simulink model "codec74"  (R2018a)
settings: Solver=VariableStepAuto  StartTime=0.0  StopTime=10.0  RelTol=1e-3
values from neighbouring files (symbols this model uses):
  pbsc74 = i    [Ejercicio44.m]
libraries: commblkcod2 x2, commrandsrc3 x1, commchan3 x1, commsink2 x1
settings Model: Creator=Alumnos  LastModifiedBy=Anselmo-PC

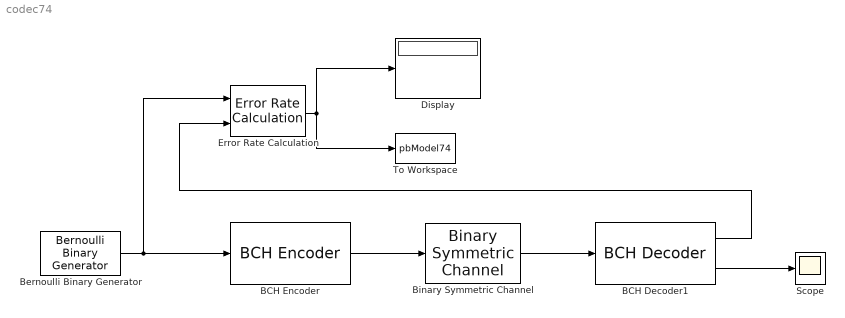
== system codec74 ==
  BCH Decoder1 : commblkcod2/BCH Decoder  n=7  k=4  specShortening=off  shortenedK=5  specGenPoly=off  genPoly='X^10 + X^8 + X^5 + X^4 + X^2 + X + 1'  specPrimPoly=off  prPoly='X^4 + X + 1'  specDisableGenCheck=off  specPuncture=off  punctVec=[ones(8,1); zeros(2,1)]  specErasurePort=off  showNumErr=on
      settings: SourceProductName=Communications System Toolbox  SourceProductBaseCode=CM
  BCH Encoder : commblkcod2/BCH Encoder  n=7  k=4  specShortening=off  shortenedK=5  specGenPoly=off  genPoly='X^10 + X^8 + X^5 + X^4 + X^2 + X + 1'  specPrimPoly=off  prPoly='X^4 + X + 1'  specDisableGenCheck=off  specPuncture=off  punctVec=[ones(8,1); zeros(2,1)]
      settings: SourceProductName=Communications System Toolbox  SourceProductBaseCode=CM
  Bernoulli Binary Generator : commrandsrc3/Bernoulli Binary Generator  ProbabilityOfZero=0.5  SeedSource=Parameter  Seed=12345  SampleTime=.00001  SamplesPerFrame=4  OutputDataType=double  SimulateUsing=Interpreted execution
  Binary Symmetric Channel : commchan3/Binary Symmetric Channel  P=pbsc74  s=2137  E=off  outDtype=double
      settings: SourceProductName=Communications System Toolbox  SourceProductBaseCode=CM
  Display : Display
  Error Rate Calculation : commsink2/Error Rate Calculation  N=0  st_delay=0  cp_mode=Entire frame  subframe=[]  PMode=Port  WsName=ErrorVec  RsMode2=off  stop=off  numErr=100  maxBits=1e6
  Scope : Scope
  To Workspace : ToWorkspace  VariableName=pbModel74  SampleTime=-1
      settings: MaxDataPoints=1
  wires:
  Bernoulli Binary Generator/1 -> Error Rate Calculation/1, BCH Encoder/1
  BCH Encoder/1 -> Binary Symmetric Channel/1
  Binary Symmetric Channel/1 -> BCH Decoder1/1
  BCH Decoder1/1 -> Error Rate Calculation/2
  BCH Decoder1/2 -> Scope/1
  Error Rate Calculation/1 -> To Workspace/1, Display/1
